simulink model "Ziegler_Nichols_closed_Loop"  (R2023b)
settings: Solver=ode3  StartTime=0.0  StopTime=30  FixedStep=0.05  RelTol=1e-3  EnableMultiTasking=on
values from neighbouring files (symbols this model uses):
  theta0 = theta    (= 4.71238898038)    [Simulation_code.m]    (also in parameters.m = -1.57079632679)
  Vmax = 0.8    [Simulation_code.m]    (also in parameters.m)
  xg = 5    [Simulation_code.m]    (also in parameters.m)
  yg = 5    [Simulation_code.m]    (also in parameters.m)
settings Model: Creator=Shaam  LastModifiedBy=Hadi
settings SolverCC: AlgebraicLoopSolver=TrustRegion
settings DataIOCC: LimitDataPoints=on  SaveFormat=Array  ReturnWorkspaceOutputs=off
settings OptimizationCC: LifeSpan=inf
settings DebuggingCC: UnderspecifiedInitializationDetection=Classic  MergeDetectMultiDrivingBlocksExec=none  SolverPrmCheckMsg=warning  UnconnectedInputMsg=warning  UnconnectedOutputMsg=warning  UnconnectedLineMsg=warning  StateNameClashWarn=warning  SFUnexpectedBacktrackingDiag=warning  SFNoUnconditionalDefaultTransitionDiag=warning  SFExecutionAtInitializationDiag=none  ArithmeticOperatorsInVariantConditions=warning
settings HardwareCC: ProdBitPerPointer=32  ProdBitPerSizeT=32  ProdBitPerPtrDiffT=32  ProdLargestAtomicFloat=None  ProdIntDivRoundTo=Undefined  ProdEndianess=Unspecified  ProdWordSize=32  ProdHWDeviceType=32-bit Generic
settings ModelReferenceCC: PropagateSignalLabelsOutOfModel=off
settings SFSimCC: SimUseLocalCustomCode=off  CustomCodeUndefinedFunction=UseInterfaceOnly
settings RTWCC: RTWUseLocalCustomCode=off
settings CodeAppCC: StateflowObjectComments=on
settings GRTTargetCC: TargetLangStandard=C89/C90 (ANSI)
settings ConfigComp: CovMetricSettings=dw  CovSaveCumulativeToWorkspaceVar=on  CovSaveSingleToWorkspaceVar=on  CovExternalEMLEnable=off

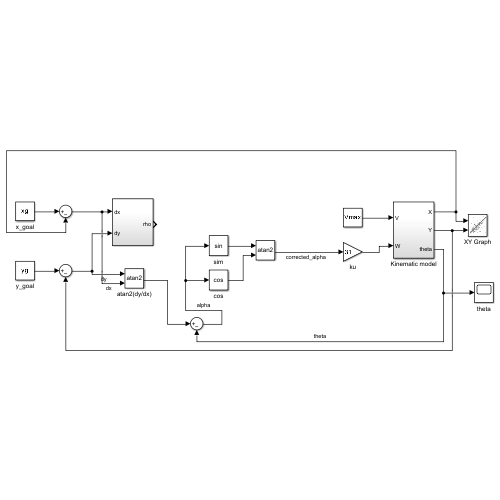
[thumbnail: Simulink's stored preview of the top-level diagram]
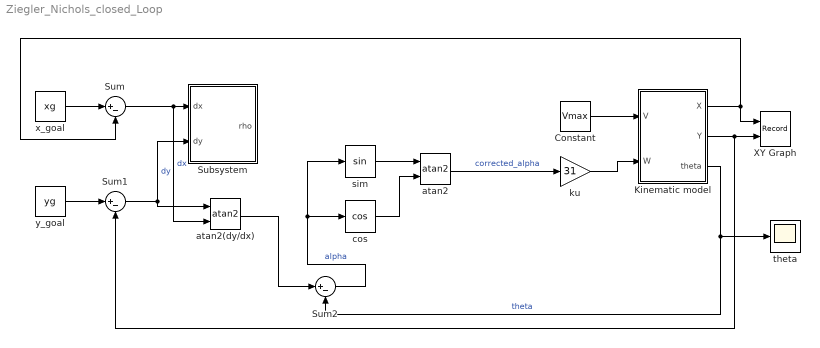
== system Ziegler_Nichols_closed_Loop ==
  Constant : Constant  Value=Vmax
  Kinematic model : Subsystem
  Subsystem : Subsystem
  Sum : Sum  Inputs=|+-
  Sum1 : Sum  Inputs=|+-
  Sum2 : Sum  Inputs=|+-
  XY Graph : Record  FileSettingsInternal="{\"entries\":[{\"content\":{\"excelSettings\":{\"content\":{},\"type\":\"Streamout.ExcelSettings\"}},\"type\":\"Streamout.FileSettingStorage\",\"uuid\":\"\"}],\"packageUris\":[\"http:\\/\\/schema.mathworks.com\\/mf0\\/streamout_blocks\\/R2020a\"],\"version\":\"1.0\"}"  Layout=[1 1]  SignalsInternal="{\"entries\":[{\"content\":{\"signals\":[{\"content\":{\"blockPath\":[],\"dimensions\":[1],\"domain\":\"\",\"lineColor\":\"#edb120\",\"port\":1,\"sid\":[\"\"],\"signalID\":542,\"signalName\":\"Kinematic model:1\"},\"type\":\"RecordBlkView.Signal\",\"uuid\":\"\"},{\"content\":{\"blockPath\":[],\"dimensions\":[1],\"domain\":\"\",\"lineColor\":\"#7e2f8e\",\"port\":2,\"sid\":[\"\"],\"signalID\":546,\"signalName\":\"Kinematic model:2\"},\"type\":\"RecordBlkView.Signal\",\"uuid\":\"\"}]},\"type\":\"RecordBlkView.InputSignals\",\"uuid\":\"\"}],\"packageUris\":[\"http:\\/\\/schema.mathworks.com\\/mf0\\/streamout_blocks\\/R2020a\"],\"version\":\"1.0\"}"  VisualizationBindings="{\"xyplotplugin\":{\"info\":[{\"series\":[],\"subplotID\":1}]}}"  CompatibilityTag=XY  st=-1
  atan2 : Trigonometry  Operator=atan2
  atan2(dy/dx) : Trigonometry  Operator=atan2
  cos : Trigonometry  Operator=cos
  ku : Gain  Gain=31
  sim : Trigonometry
  theta : Scope
  x_goal : Constant  Value=xg
  y_goal : Constant  Value=yg
  wires:
  Kinematic model/1(X) -> XY Graph/1, Sum/2
  Kinematic model/2(Y) -> XY Graph/2, Sum1/2
  Kinematic model/3(theta) -> theta/1, Sum2/2  "theta"
  x_goal/1 -> Sum/1
  y_goal/1 -> Sum1/1
  Sum1/1 -> Subsystem/2(dy), atan2(dy/dx)/1  "dy"
  Sum/1 -> atan2(dy/dx)/2, Subsystem/1(dx)  "dx"
  Sum2/1 -> cos/1, sim/1  "alpha"
  ku/1 -> Kinematic model/2(W)
  Constant/1 -> Kinematic model/1(V)
  sim/1 -> atan2/1
  cos/1 -> atan2/2
  atan2/1 -> ku/1  "corrected_alpha"
  atan2(dy/dx)/1 -> Sum2/1

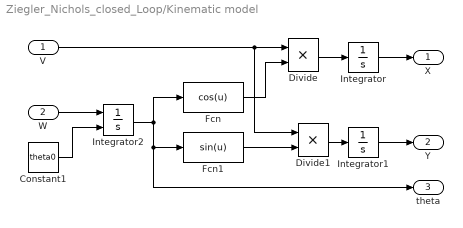
== system Ziegler_Nichols_closed_Loop/Kinematic model ==
  V : Inport
  W : Inport  Port=2
  Constant1 : Constant  Value=theta0
  Divide : Product  Inputs=**
  Divide1 : Product  Inputs=**
  Fcn : Fcn  Expr=cos(u)
  Fcn1 : Fcn  Expr=sin(u)
  Integrator : Integrator
  Integrator1 : Integrator
  Integrator2 : Integrator  InitialConditionSource=external
  X : Outport
  Y : Outport  Port=2
  theta : Outport  Port=3
  wires:
  V/1 -> Divide1/1, Divide/1
  W/1 -> Integrator2/1
  Integrator2/1 -> theta/1, Fcn1/1, Fcn/1
  Divide1/1 -> Integrator1/1
  Fcn/1 -> Divide/2
  Divide/1 -> Integrator/1
  Integrator1/1 -> Y/1
  Integrator/1 -> X/1
  Fcn1/1 -> Divide1/2
  Constant1/1 -> Integrator2/2

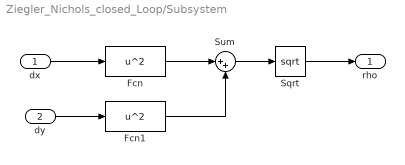
== system Ziegler_Nichols_closed_Loop/Subsystem ==
  dx : Inport
  dy : Inport  Port=2
  Fcn : Fcn  Expr=u^2
  Fcn1 : Fcn  Expr=u^2
  Sqrt : Sqrt
  Sum : Sum  Inputs=|++
  rho : Outport
  wires:
  dy/1 -> Fcn1/1
  Sqrt/1 -> rho/1
  Fcn1/1 -> Sum/2
  Fcn/1 -> Sum/1
  Sum/1 -> Sqrt/1
  dx/1 -> Fcn/1
